simulink model "Ques_3_3_PendulumModel"  (R2020a)
settings: Solver=VariableStepAuto  StartTime=0.0  StopTime=100  RelTol=1e-3
settings Model: Creator=UtelPhone  LastModifiedBy=UtelPhone

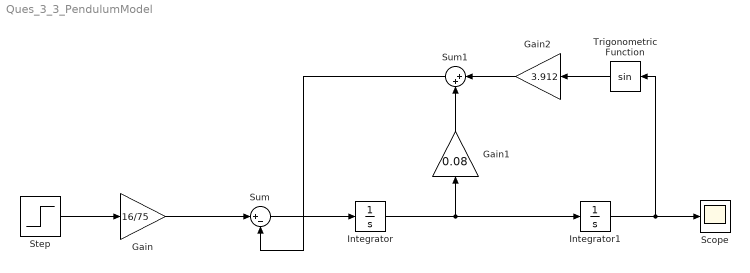
== system Ques_3_3_PendulumModel ==
  Gain : Gain  Gain=16/75
  Gain1 : Gain  Gain=0.08
  Gain2 : Gain  Gain=3.912
  Integrator : Integrator
  Integrator1 : Integrator
  Scope : Scope
  Step : Step  Time=0  After=200  SampleTime=0
  Sum : Sum  Inputs=|+-
  Sum1 : Sum  Inputs=|++
  Trigonometric Function : Trigonometry
  wires:
  Gain/1 -> Sum/1
  Step/1 -> Gain/1
  Sum/1 -> Integrator/1
  Integrator/1 -> Integrator1/1, Gain1/1
  Gain1/1 -> Sum1/2
  Gain2/1 -> Sum1/1
  Trigonometric Function/1 -> Gain2/1
  Integrator1/1 -> Scope/1, Trigonometric Function/1
  Sum1/1 -> Sum/2
